simulink subsystem "debug_publisher"  (R2025b)
settings: Solver=VariableStepAuto  StartTime=0.0  StopTime=10.0  RelTol=1e-3
undefined symbols (not defined in the file or in its folder): dt_debug
libraries: ros2lib x2
settings Model: Creator=kjhaydon  LastModifiedBy=kjhaydon

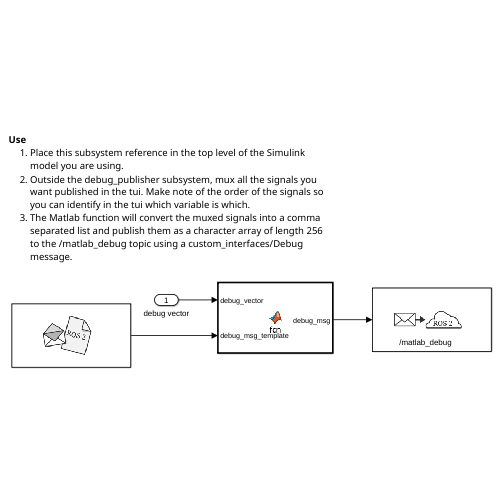
[thumbnail: Simulink's stored preview of the top-level diagram]
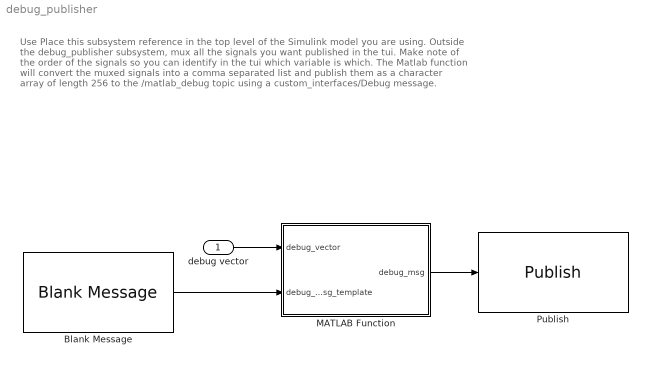
== system debug_publisher ==
  note: Use
      | Place this subsystem reference in the top level of the Simulink model you are using.
      | Outside the debug_publisher subsystem, mux all the signals you want published in the tui. Make note of the order of the signals so you can identify in the tui which variable is which.
      | The Matlab function will convert the muxed signals into a comma separated list and publish them as a character array of length 256 to the /matlab_debug topic using a custom_interfaces/Debug message.
  debug vector : Inport  SampleTime=dt_debug
  Blank Message : ros2lib/Blank Message  messageClass=Message  entityType=custom_interfaces/Debug  messageType=custom_interfaces/Debug  SampleTime=inf
  MATLAB Function : MATLAB Function  TreatAsAtomicUnit=on
  Publish : ros2lib/Publish  topicSource=Specify your own  topic=/matlab_debug  messageType=geometry_msgs/Point  QOSHistory=Keep last  QOSDepth=10  QOSReliability=Reliable  QOSDurability=Volatile  QOSDeadline=Inf  QOSLifespan=Inf  QOSLiveliness=Automatic  QOSLeaseDuration=Inf  QOSAvoidROSNamespaceConventions=off
  wires:
  debug vector/1 -> MATLAB Function/1(debug_vector)
  Blank Message/1 -> MATLAB Function/2(debug_msg_template)
  MATLAB Function/1(debug_msg) -> Publish/1

== matlab function debug_publisher/MATLAB Function ==
  data: debug_vector input; debug_msg output SL_Bus_custom_interfaces_Debug; debug_msg_template input SL_Bus_custom_interfaces_Debug
function debug_msg = fcn(debug_vector, debug_msg_template)

%{
This function converts the debug_vector to a comma separated list, pads or
trims it to 256 characters, then packs it into a
SL_Bus_custom_interfaces_Debug bus for publishing. 

Make sure the data type for the input debug_msg_template and the output
debug_msg is set to SL_Bus_custom_interfaces_Debug. If it is not showing up
as a valid option, use ros.ros2.createSimulinkBus(gcs) in the command
window.
%}
debug_msg = debug_msg_template; %initialize message to the blank template

temp_string = ""; %string for easier manipulation


for k = 1:length(debug_vector)
    temp_string = temp_string + string(debug_vector(k));
    %add commas between every value except at the end
    if(k < length(debug_vector))
        temp_string = temp_string + ",";
    end

end
temp_char = char(temp_string);
%if the array is too short, pad it to 256
while(length(temp_char) < 256)
    temp_char = [temp_char,'_'];
end
%if the array is too long, trim it to 256
if(length(temp_char) > 256)
    temp_char = temp_char(1:256);
end

%temp char is gauranteed to be of length 256 now, so we can pack it into
%the debug message
debug_msg.data = temp_char;
